simulink library "NG_CHP_lib"  (Simulink 8.1)
settings: Solver=ode45  StartTime=0.0  StopTime=10.0  RelTol=1e-3
undefined symbols (not defined in the file): fdesignblkfcn, gcbh, ph, SIM_HIL, Ts
libraries: simulink x23, rtio_opalrt_common x21, simulink_extras x6, rteventslib x4, CHP_Model_lib x1, NG_Genset_lib x1, rtio_generic_modbus x1
(part 1 of 2)
settings Model: Creator=re25624  LastModifiedBy=re25624

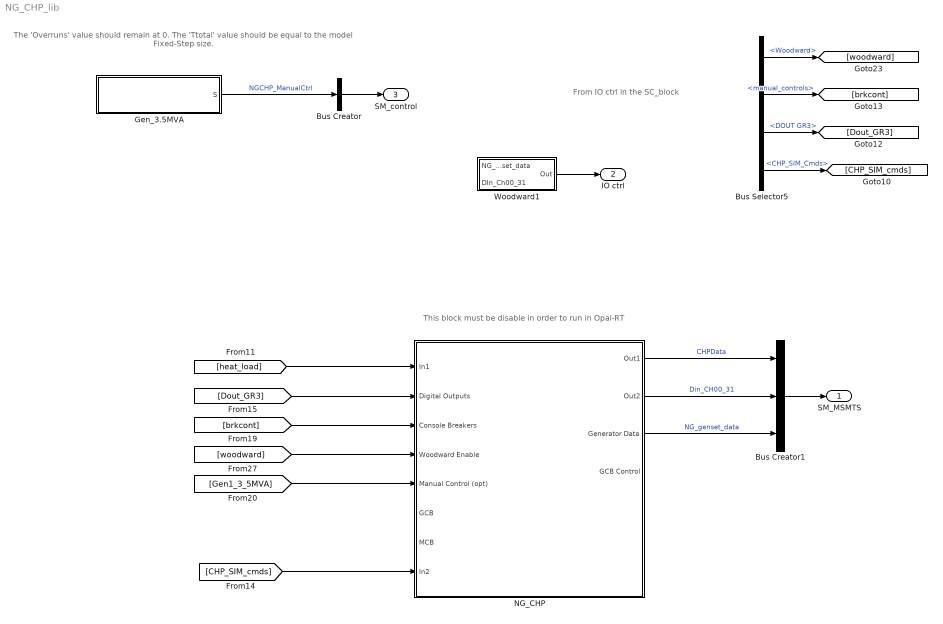
== system NG_CHP_lib ==
  note: From IO ctrl in the SC_block
  note: This block must be disable in order to run in Opal-RT
  note: The 'Overruns' value should remain at 0.
      | The 'Ttotal' value should be equal to the
      | model Fixed-Step size.
  Bus Creator : BusCreator  Inputs=1
  Bus Creator1 : BusCreator  Inputs=3
  Bus Selector5 : BusSelector  OutputSignals=Woodward,manual_controls,DOUT GR3,DOUT GR3.16 DOUT GR3.CHP_SIM_Cmds
  Gen_3.5MVA : Subsystem
  NG_CHP : Subsystem
  Woodward1 : Subsystem
  SM_MSMTS : Outport
  IO ctrl : Outport  Port=2
  SM_control : Outport  Port=3
  wires:
  [Dout_GR3] -> NG_CHP/2(Digital Outputs)
  [brkcont] -> NG_CHP/3(Console Breakers)
  [woodward] -> NG_CHP/4(Woodward Enable)
  [Gen1_3_5MVA] -> NG_CHP/5(Manual Control (opt))
  [heat_load] -> NG_CHP/1(In1)
  Bus Creator1/1 -> SM_MSMTS/1
  NG_CHP/3(Generator Data) -> Bus Creator1/3  "NG_genset_data"
  NG_CHP/2(Out2) -> Bus Creator1/2  "Din_CH00_31"
  NG_CHP/1(Out1) -> Bus Creator1/1  "CHPData"
  [CHP_SIM_cmds] -> NG_CHP/8(In2)
  ? -> Bus Selector5/1
  Bus Selector5/1 -> [woodward]  "<Woodward>"
  Bus Selector5/3 -> [Dout_GR3]  "<DOUT GR3>"
  Bus Selector5/2 -> [brkcont]  "<manual_controls>"
  Bus Selector5/4 -> [CHP_SIM_cmds]  "<CHP_SIM_Cmds>"
  Woodward1/1(Out) -> IO ctrl/1
  Gen_3.5MVA/1(S) -> Bus Creator/1  "NGCHP_ManualCtrl"
  Bus Creator/1 -> SM_control/1

== system NG_CHP_lib/Gen_3.5MVA ==
  1 - PQ 2 - PV 3 - VF : Constant  Value=3
  2.5 - 130 s : DiscretePulseGenerator  Period=150/Ts  PulseWidth=127.5/Ts  PhaseDelay=2.5/Ts  SampleTime=Ts
  Bus Creator : BusCreator  Inputs=6
  DONOTCHANGE : Constant
  Enable = 1 Disable = 0 : Constant  Value=0
  F : simulink/Math Operations/Slider Gain  low=0.97  gain=1  high=1.03
  Fcmd pu : Constant  Value=1.0
  P : simulink/Math Operations/Slider Gain  low=0  gain=0.8  high=1.1
  Pfactor : Gain  Gain=.9
  Q : simulink/Math Operations/Slider Gain  low=0.01  gain=0.2  high=0.4
  Qfactor : Gain  Gain=.43
  S Profile : simulink/Sources/Repeating Sequence Stair  OutValues=[.1 .1 .1 .1 .1 .1 .5 .5 .5 .5 .5 .5 .5 .5 .5 .5 .5 .5 1 1 1 1 1 ]  tsamp=[5 Ts]  OutMin=[]  OutMax=[]  OutDataTypeStr=Inherit: Inherit via back propagation  OutDataType=fixdt(0,8)  ConRadixGroup=Best Precision: Vector-wise  OutScaling=2^-12
  V : simulink/Math Operations/Slider Gain  low=0.9  gain=1  high=1.1
  VF - to end : simulink/Sources/Repeating Sequence Stair  OutValues=[3 3 3 3 3 3 3 3 3 3 3 3 3 3 3 3 3 3 3 3 3 3 3 3 3 3 3 3 3 3 3 ]  tsamp=[5 Ts]  OutMin=[]  OutMax=[]  OutDataTypeStr=Inherit: Inherit via back propagation  OutDataType=fixdt(0,8)  ConRadixGroup=Best Precision: Vector-wise  OutScaling=2^-12
  Vcmd pu : Constant
  S : Outport
  wires:
  DONOTCHANGE/1 -> P/1, Q/1, V/1, F/1
  Bus Creator/1 -> S/1
  S Profile/1 -> Qfactor/1, Pfactor/1  "P"
  Qfactor/1 -> Bus Creator/2  "Q"
  Vcmd pu/1 -> Bus Creator/3  "V"
  VF - to end/1 -> Bus Creator/5  "Mode"
  2.5 - 130 s/1 -> Bus Creator/6  "Enable"
  Fcmd pu/1 -> Bus Creator/4  "F"
  Pfactor/1 -> Bus Creator/1  "P"

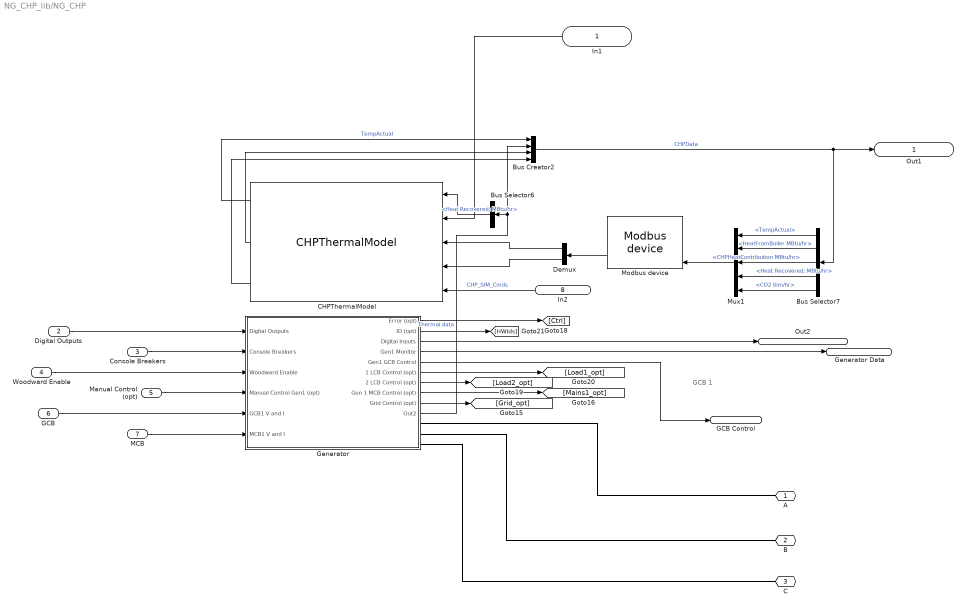
== system NG_CHP_lib/NG_CHP ==
  note: GCB 1
  In1 : Inport
  Digital Outputs : Inport  Port=2
  Console Breakers : Inport  Port=3
  Woodward Enable : Inport  Port=4
  Manual Control (opt) : Inport  Port=5
  GCB : Inport  Port=6
  MCB : Inport  Port=7
  In2 : Inport  Port=8
  Bus Creator2 : BusCreator
  Bus Selector6 : BusSelector  OutputSignals=Heat Recovered; MBtu/hr
  Bus Selector7 : BusSelector  OutputSignals=TempActual,HeatFromBoiler MBtu/hr,CHPHeatContribution MBtu/hr,Thermal data.Heat Recovered; MBtu/hr,Thermal data.CO2 lbm/hr
  CHPThermalModel : CHP_Model_lib/CHPThermalModel  SIM_HIL=SIM_HIL
  Demux : Demux  Outputs=2
  Generator : Subsystem  AncestorBlock=NG_Genset_lib/Generator
  Modbus device : rtio_generic_modbus/Modbus device  conf_name=CHP_slave_cfg.opal  conf_name_mask=CHP_slave_cfg.xls  sample_time=Ts
  Mux1 : Mux  Inputs=5
  A : PMIOPort  Tag=A  Port=1  Side=Right
      settings: AttributesFormatString=A
  B : PMIOPort  Port=2  Side=Right
  C : PMIOPort  Port=3  Side=Right
  Out1 : Outport
  Out2 : Outport  Port=2
  Generator Data : Outport  Port=3
  GCB Control : Outport  Port=4
  wires:
  In2/1 -> CHPThermalModel/5  "CHP_SIM_Cmds"
  Generator/3(Digital Inputs) -> Out2/1
  Bus Creator2/1 -> Out1/1, Bus Selector7/1  "CHPData"
  Bus Selector6/1 -> CHPThermalModel/1  "<Heat Recovered; MBtu/hr>"
  Generator/6(1 LCB Control (opt)) -> [Load1_opt]
  Generator/5(Gen1 GCB Control) -> GCB Control/1
  MCB/1 -> Generator/6(MCB1 V and I)
  Generator/7(2 LCB Control (opt)) -> [Load2_opt]
  Manual Control (opt)/1 -> Generator/4(Manual Control Gen1 (opt))
  GCB/1 -> Generator/5(GCB1 V and I)
  Generator/4(Gen1 Monitor) -> Generator Data/1
  Generator/1(Error (opt)) -> [Ctrl]
  Woodward Enable/1 -> Generator/3(Woodward Enable)
  Generator/2(ID (opt)) -> [HWIds]
  Modbus device/2 -> Demux/1
  Generator/10(Out2) -> Bus Selector6/1, Bus Creator2/2  "Thermal data"
  CHPThermalModel/3 -> Bus Creator2/4
  Demux/1 -> CHPThermalModel/3
  Mux1/1 -> Modbus device/4
  In1/1 -> CHPThermalModel/2
  Bus Selector7/1 -> Mux1/1  "<TempActual>"
  Bus Selector7/4 -> Mux1/4  "<Heat Recovered; MBtu/hr>"
  Bus Selector7/5 -> Mux1/5  "<CO2 lbm/hr>"
  Bus Selector7/2 -> Mux1/2  "<HeatFromBoiler MBtu/hr>"
  Digital Outputs/1 -> Generator/1(Digital Outputs)
  Generator/9(Grid Control (opt)) -> [Grid_opt]
  Console Breakers/1 -> Generator/2(Console Breakers)
  Generator/8(Gen 1 MCB Control (opt)) -> [Mains1_opt]
  CHPThermalModel/2 -> Bus Creator2/3
  Demux/2 -> CHPThermalModel/4
  CHPThermalModel/1 -> Bus Creator2/1  "TempActual"
  Bus Selector7/3 -> Mux1/3  "<CHPHeatContribution MBtu/hr>"
  connections:
  Generator/RConn1 -- A/RConn1
  Generator/RConn2 -- B/RConn1
  Generator/RConn3 -- C/RConn1

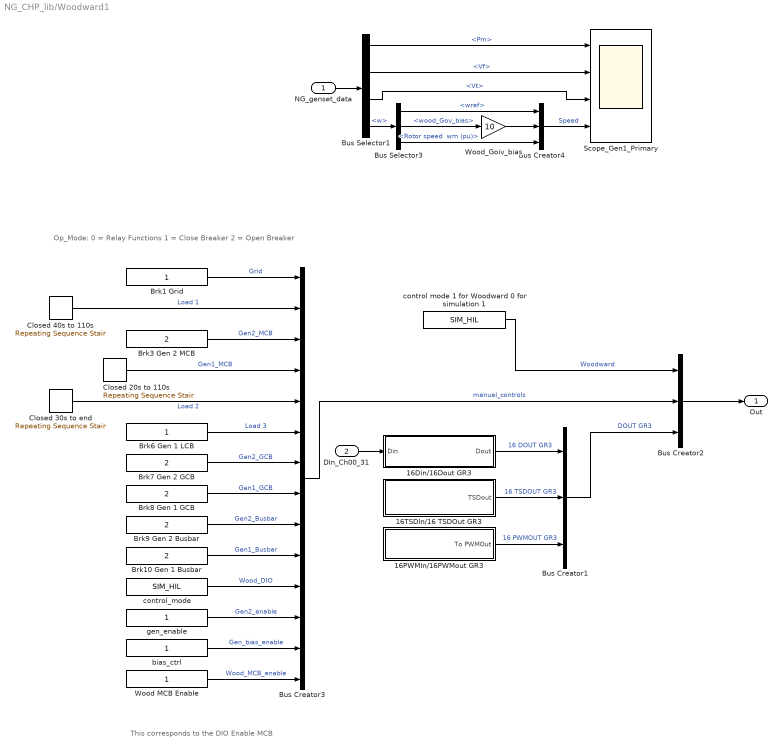
== system NG_CHP_lib/Woodward1 ==
  note: Op_Mode:
      | 0 = Relay Functions
      | 1 = Close Breaker
      | 2 = Open Breaker
  note: This corresponds to
      | the DIO Enable MCB
  NG_genset_data : Inport
  DIn_Ch00_31 : Inport  Port=2
  16Din/16Dout GR3 : Subsystem
  16PWMIn/16PWMout GR3 : Subsystem
  16TSDIn/16 TSDOut GR3 : Subsystem
  Brk1 Grid : Constant
  Brk10 Gen 1 Busbar : Constant  Value=2
  Brk3 Gen 2 MCB : Constant  Value=2
  Brk6 Gen 1 LCB : Constant
  Brk7 Gen 2 GCB : Constant  Value=2
  Brk8 Gen 1 GCB : Constant  Value=2
  Brk9 Gen 2 Busbar : Constant  Value=2
  Bus Creator1 : BusCreator  Inputs=3
  Bus Creator2 : BusCreator  Inputs=3
  Bus Creator3 : BusCreator  Inputs=14
  Bus Creator4 : BusCreator  Inputs=3
  Bus Selector1 : BusSelector  OutputSignals=Pm,Vf,Vt,w
  Bus Selector3 : BusSelector  OutputSignals="wref,w.wood_Gov_bias,w.Rotor speed  wm (pu)"
  Closed 20s to 110s : simulink/Sources/Repeating Sequence Stair  OutValues=[2 2 2 2 1 1 1 1 1 1 1 1 1 1 1 1 1 1 1 1 1 1 2 2 2 2 2]  tsamp=[5 Ts]  OutMin=[]  OutMax=[]  OutDataTypeStr=double  OutputDataTypeScalingMode=double  OutDataType=fixdt(0,8)  ConRadixGroup=Best Precision: Vector-wise  OutScaling=2^-12
  Closed 30s to end : simulink/Sources/Repeating Sequence Stair  OutValues=[2 2 2 2 2 2 1 1 1 1 1 1 1 1 1 1 1 1 1 1 1 1 ]  tsamp=[5 Ts]  OutMin=[]  OutMax=[]  OutDataTypeStr=double  OutputDataTypeScalingMode=double  OutDataType=fixdt(0,8)  ConRadixGroup=Best Precision: Vector-wise  OutScaling=2^-12
  Closed 40s to 110s : simulink/Sources/Repeating Sequence Stair  OutValues=[2 2 2 2 2 2 2 2 1 1 1 1 1 1 1 1 1 1 1 1 1 1 2 2 2]  tsamp=[5 Ts]  OutMin=[]  OutMax=[]  OutDataTypeStr=double  OutputDataTypeScalingMode=double  OutDataType=fixdt(0,8)  ConRadixGroup=Best Precision: Vector-wise  OutScaling=2^-12
  Scope_Gen1_Primary : Scope  NumInputPorts=4
      settings: TimeRange=10  YMin=-0.05~-0.5~0~0  YMax=0.8~5.5~1.1~1.1  SaveName=ScopeData4
  Wood MCB Enable : Constant
  Wood_Goiv_bias : Gain  Gain=10
  bias_ctrl : Constant
  control mode 1 for Woodward 0 for simulation 1 : Constant  Value=SIM_HIL
  control_mode : Constant  Value=SIM_HIL
  gen_enable : Constant
  Out : Outport
  wires:
  control mode 1 for Woodward 0 for simulation 1/1 -> Bus Creator2/1  "Woodward"
  16Din/16Dout GR3/1(Dout) -> Bus Creator1/1  "16 DOUT GR3"
  16TSDIn/16 TSDOut GR3/1(TSDout) -> Bus Creator1/2  "16 TSDOUT GR3"
  16PWMIn/16PWMout GR3/1(To PWMOut) -> Bus Creator1/3  "16 PWMOUT GR3"
  Bus Creator1/1 -> Bus Creator2/3  "DOUT GR3"
  Bus Creator3/1 -> Bus Creator2/2  "manual_controls"
  Closed 40s to 110s/1 -> Bus Creator3/2  "Load 1"
  Brk3 Gen 2 MCB/1 -> Bus Creator3/3  "Gen2_MCB"
  Closed 20s to 110s/1 -> Bus Creator3/4  "Gen1_MCB"
  control_mode/1 -> Bus Creator3/11  "Wood_DIO"
  gen_enable/1 -> Bus Creator3/12  "Gen2_enable"
  bias_ctrl/1 -> Bus Creator3/13  "Gen_bias_enable"
  Bus Creator2/1 -> Out/1
  DIn_Ch00_31/1 -> 16Din/16Dout GR3/1(Din)
  Bus Selector1/1 -> Scope_Gen1_Primary/1  "<Pm>"
  Bus Selector1/2 -> Scope_Gen1_Primary/2  "<Vf>"
  Bus Selector1/3 -> Scope_Gen1_Primary/3  "<Vt>"
  NG_genset_data/1 -> Bus Selector1/1
  Wood MCB Enable/1 -> Bus Creator3/14  "Wood_MCB_enable"
  Bus Selector1/4 -> Bus Selector3/1  "<w>"
  Bus Selector3/1 -> Bus Creator4/1  "<wref>"
  Bus Selector3/2 -> Wood_Goiv_bias/1  "<wood_Gov_bias>"
  Bus Selector3/3 -> Bus Creator4/3  "<Rotor speed  wm (pu)>"
  Bus Creator4/1 -> Scope_Gen1_Primary/4  "Speed"
  Closed 30s to end/1 -> Bus Creator3/5  "Load 2"
  Brk6 Gen 1 LCB/1 -> Bus Creator3/6  "Load 3"
  Brk7 Gen 2 GCB/1 -> Bus Creator3/7  "Gen2_GCB"
  Brk8 Gen 1 GCB/1 -> Bus Creator3/8  "Gen1_GCB"
  Wood_Goiv_bias/1 -> Bus Creator4/2
  Brk9 Gen 2 Busbar/1 -> Bus Creator3/9  "Gen2_Busbar"
  Brk10 Gen 1 Busbar/1 -> Bus Creator3/10  "Gen1_Busbar"
  Brk1 Grid/1 -> Bus Creator3/1  "Grid"

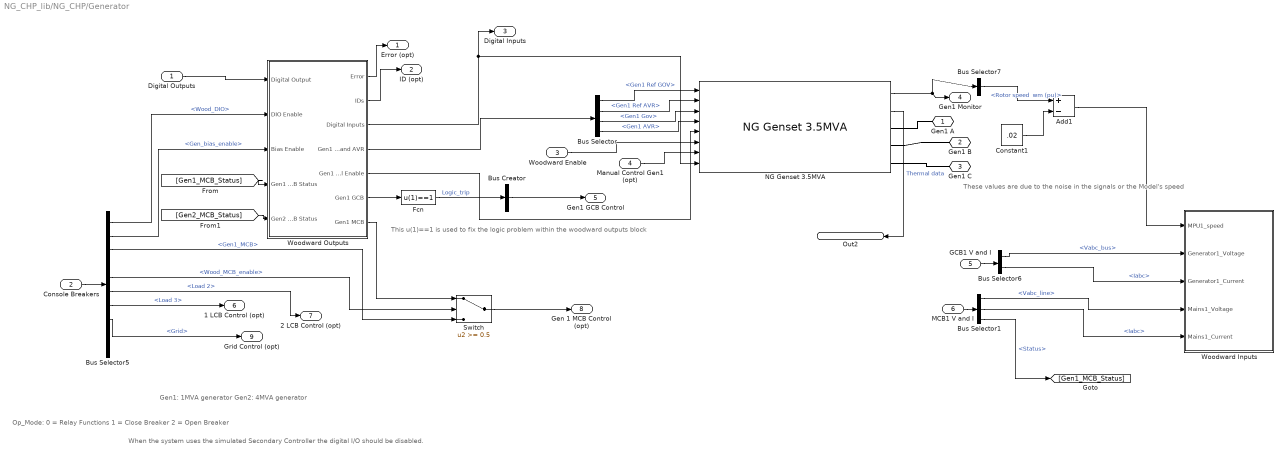
== system NG_CHP_lib/NG_CHP/Generator ==
  note: Op_Mode:
      | 0 = Relay Functions
      | 1 = Close Breaker
      | 2 = Open Breaker
  note: These values are due to
      | the noise in the signals
      | or the Model's speed
  note: Gen1: 1MVA generator
      | Gen2: 4MVA generator
  note: When the system uses the simulated
      | Secondary Controller the digital I/O
      | should be disabled.
  note: This u(1)==1 is used to fix the logic problem within the woodward outputs block
  Digital Outputs : Inport
  Console Breakers : Inport  Port=2
  Woodward Enable : Inport  Port=3
  Manual Control Gen1 (opt) : Inport  Port=4
  GCB1 V and I : Inport  Port=5
  MCB1 V and I : Inport  Port=6
  Add1 : Sum  Inputs=+-
  Bus Creator : BusCreator  Inputs=1
  Bus Selector : BusSelector  OutputSignals=Gen1 Ref GOV,Gen1 Ref AVR,Gen1 Gov,Gen1 AVR
  Bus Selector1 : BusSelector  OutputSignals=Vabc_line,Iabc,Status
  Bus Selector5 : BusSelector  OutputSignals=Wood_DIO,Gen_bias_enable,Gen1_MCB,Gen2_MCB,Wood_MCB_enable,Load 2,Load 3,Grid,Gen2_enable,Load 1
  Bus Selector6 : BusSelector  OutputSignals=Vabc_bus,Iabc
  Bus Selector7 : BusSelector  OutputSignals="w.w.Rotor speed  wm (pu)"
  Constant1 : Constant  Value=.02
  Fcn : Fcn  Expr=u(1)==1
  NG Genset 3.5MVA : NG_Genset_lib/NG Genset 3.5MVA  control_mode=1
  Switch : Switch  Threshold=0.5
  Woodward Inputs : Subsystem
  Woodward Outputs : Subsystem
  Gen1 A : PMIOPort  Port=1  Side=Right
  Gen1 B : PMIOPort  Port=2  Side=Right
  Gen1 C : PMIOPort  Port=3  Side=Right
  Error (opt) : Outport
  ID (opt) : Outport  Port=2
  Digital Inputs : Outport  Port=3
  Gen1 Monitor : Outport  Port=4
  Gen1 GCB Control : Outport  Port=5
  1 LCB Control (opt) : Outport  Port=6
  2 LCB Control (opt) : Outport  Port=7
  Gen 1 MCB Control (opt) : Outport  Port=8
  Grid Control (opt) : Outport  Port=9
  Out2 : Outport  Port=10
  wires:
  Fcn/1 -> Bus Creator/1  "Logic_trip"
  Bus Creator/1 -> Gen1 GCB Control/1
  NG Genset 3.5MVA/1 -> Bus Selector7/1, Gen1 Monitor/1
  Bus Selector6/1 -> Woodward Inputs/2(Generator1_Voltage)  "<Vabc_bus>"
  Bus Selector6/2 -> Woodward Inputs/3(Generator1_Current)  "<Iabc>"
  Bus Selector5/1 -> Woodward Outputs/2(DIO Enable)  "<Wood_DIO>"
  Manual Control Gen1 (opt)/1 -> NG Genset 3.5MVA/7
  Bus Selector5/2 -> Woodward Outputs/3(Bias Enable)  "<Gen_bias_enable>"
  Bus Selector7/1 -> Add1/1  "<Rotor speed  wm (pu)>"
  Woodward Outputs/1(Error) -> Error (opt)/1
  Woodward Outputs/2(IDs) -> ID (opt)/1
  Woodward Enable/1 -> NG Genset 3.5MVA/6
  Woodward Outputs/5(Gen1 Fuel Enable) -> NG Genset 3.5MVA/5
  Bus Selector5/5 -> Switch/2  "<Wood_MCB_enable>"
  Woodward Outputs/7(Gen1 MCB) -> Switch/1
  Digital Outputs/1 -> Woodward Outputs/1(Digital Output)
  GCB1 V and I/1 -> Bus Selector6/1
  Woodward Outputs/6(Gen1 GCB) -> Fcn/1
  Console Breakers/1 -> Bus Selector5/1
  Bus Selector5/7 -> 1 LCB Control (opt)/1  "<Load 3>"
  Switch/1 -> Gen 1 MCB Control (opt)/1
  MCB1 V and I/1 -> Bus Selector1/1
  Bus Selector1/1 -> Woodward Inputs/4(Mains1_Voltage)  "<Vabc_line>"
  Bus Selector1/2 -> Woodward Inputs/5(Mains1_Current)  "<Iabc>"
  Woodward Outputs/4(Gen1 Gov and AVR) -> Bus Selector/1
  Bus Selector/1 -> NG Genset 3.5MVA/1  "<Gen1 Ref GOV>"
  Bus Selector/2 -> NG Genset 3.5MVA/2  "<Gen1 Ref AVR>"
  Bus Selector/3 -> NG Genset 3.5MVA/3  "<Gen1 Gov>"
  Bus Selector/4 -> NG Genset 3.5MVA/4  "<Gen1 AVR>"
  Bus Selector1/3 -> [Gen1_MCB_Status]  "<Status>"
  [Gen1_MCB_Status] -> Woodward Outputs/4(Gen1 MCB Status)
  [Gen2_MCB_Status] -> Woodward Outputs/5(Gen2 MCB Status)
  Bus Selector5/6 -> 2 LCB Control (opt)/1  "<Load 2>"
  Bus Selector5/3 -> Switch/3  "<Gen1_MCB>"
  Bus Selector5/8 -> Grid Control (opt)/1  "<Grid>"
  Constant1/1 -> Add1/2
  NG Genset 3.5MVA/2 -> Out2/1  "Thermal data"
  Add1/1 -> Woodward Inputs/1(MPU1_speed)
  Woodward Outputs/3(Digital Inputs) -> Digital Inputs/1, NG Genset 3.5MVA/8
  connections:
  NG Genset 3.5MVA/RConn1 -- Gen1 A/RConn1
  NG Genset 3.5MVA/RConn2 -- Gen1 B/RConn1
  NG Genset 3.5MVA/RConn3 -- Gen1 C/RConn1

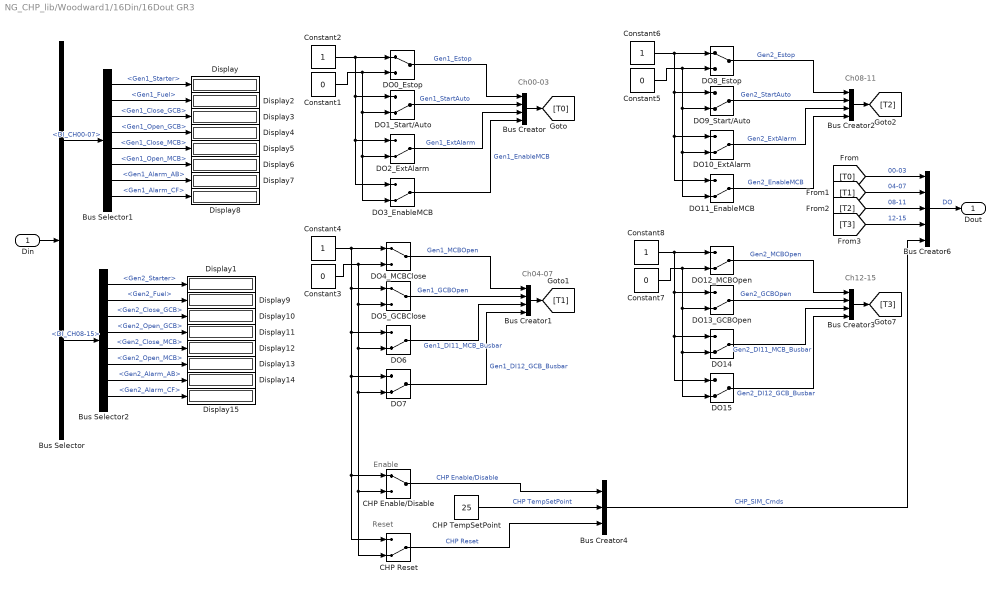
== system NG_CHP_lib/Woodward1/16Din/16Dout GR3 ==
  note: Ch00-03
  note: Ch04-07
  note: Ch08-11
  note: Ch12-15
  note: Enable
  note: Reset
  Din : Inport
  Bus Creator{,1..3} (4 alike) : BusCreator
  Bus Creator4 : BusCreator  Inputs=3
  Bus Creator6 : BusCreator  Inputs=5
  Bus Selector : BusSelector  OutputSignals=DIN.DI_CH00-07,DIN.DI_CH08-15
  Bus Selector1 : BusSelector  OutputSignals=Gen1_Starter,Gen1_Fuel,Gen1_Close_GCB,Gen1_Open_GCB,Gen1_Close_MCB,Gen1_Open_MCB,Gen1_Alarm_AB,Gen1_Alarm_CF
  Bus Selector2 : BusSelector  OutputSignals=Gen2_Starter,Gen2_Fuel,Gen2_Close_GCB,Gen2_Open_GCB,Gen2_Close_MCB,Gen2_Open_MCB,Gen2_Alarm_AB,Gen2_Alarm_CF
  CHP Enable/Disable : ManualSwitch
  CHP Reset : ManualSwitch  CurrentSetting=0
  CHP TempSetPoint : Constant  Value=25
  Constant{1,3,5,7} (4 alike) : Constant  Value=0
  Constant{2,4,6,8} (4 alike) : Constant
  DO0_Estop : ManualSwitch
  DO10_ExtAlarm : ManualSwitch  CurrentSetting=0
  DO11_EnableMCB : ManualSwitch  CurrentSetting=0
  DO12_MCBOpen : ManualSwitch  CurrentSetting=0
  DO13_GCBOpen : ManualSwitch  CurrentSetting=0
  DO{6..7,14..15} (4 alike) : ManualSwitch  CurrentSetting=0
  DO1_Start/Auto : ManualSwitch  CurrentSetting=0
  DO2_ExtAlarm : ManualSwitch  CurrentSetting=0
  DO3_EnableMCB : ManualSwitch  CurrentSetting=0
  DO4_MCBClose : ManualSwitch
  DO5_GCBClose : ManualSwitch
  DO8_Estop : ManualSwitch
  DO9_Start/Auto : ManualSwitch  CurrentSetting=0
  Display{,1..15} (16 alike) : Display
  Dout : Outport
  wires:
  Bus Creator4/1 -> Bus Creator6/5  "CHP_SIM_Cmds"
  CHP Reset/1 -> Bus Creator4/3  "CHP Reset"
  CHP TempSetPoint/1 -> Bus Creator4/2  "CHP TempSetPoint"
  CHP Enable/Disable/1 -> Bus Creator4/1  "CHP Enable/Disable"
  Bus Creator6/1 -> Dout/1  "DO"
  Constant2/1 -> DO0_Estop/1, DO1_Start/Auto/1, DO3_EnableMCB/1, DO2_ExtAlarm/1
  Constant1/1 -> DO0_Estop/2, DO1_Start/Auto/2, DO3_EnableMCB/2, DO2_ExtAlarm/2
  DO0_Estop/1 -> Bus Creator/1  "Gen1_Estop"
  DO1_Start/Auto/1 -> Bus Creator/2  "Gen1_StartAuto"
  DO2_ExtAlarm/1 -> Bus Creator/3  "Gen1_ExtAlarm"
  DO3_EnableMCB/1 -> Bus Creator/4  "Gen1_EnableMCB"
  Constant4/1 -> DO6/1, DO7/1, CHP Enable/Disable/1, CHP Reset/1, DO5_GCBClose/1, DO4_MCBClose/1
  Constant3/1 -> DO6/2, CHP Enable/Disable/2, CHP Reset/2, DO7/2, DO5_GCBClose/2, DO4_MCBClose/2
  DO4_MCBClose/1 -> Bus Creator1/1  "Gen1_MCBOpen"
  DO5_GCBClose/1 -> Bus Creator1/2  "Gen1_GCBOpen"
  DO6/1 -> Bus Creator1/3  "Gen1_DI11_MCB_Busbar"
  DO7/1 -> Bus Creator1/4  "Gen1_DI12_GCB_Busbar"
  Constant6/1 -> DO8_Estop/1, DO9_Start/Auto/1, DO11_EnableMCB/1, DO10_ExtAlarm/1
  Constant5/1 -> DO8_Estop/2, DO9_Start/Auto/2, DO11_EnableMCB/2, DO10_ExtAlarm/2
  DO8_Estop/1 -> Bus Creator2/1  "Gen2_Estop"
  DO9_Start/Auto/1 -> Bus Creator2/2  "Gen2_StartAuto"
  DO10_ExtAlarm/1 -> Bus Creator2/3  "Gen2_ExtAlarm"
  DO11_EnableMCB/1 -> Bus Creator2/4  "Gen2_EnableMCB"
  Constant8/1 -> DO14/1, DO15/1, DO13_GCBOpen/1, DO12_MCBOpen/1
  Constant7/1 -> DO14/2, DO15/2, DO13_GCBOpen/2, DO12_MCBOpen/2
  DO12_MCBOpen/1 -> Bus Creator3/1  "Gen2_MCBOpen"
  DO13_GCBOpen/1 -> Bus Creator3/2  "Gen2_GCBOpen"
  DO14/1 -> Bus Creator3/3  "Gen2_DI11_MCB_Busbar"
  DO15/1 -> Bus Creator3/4  "Gen2_DI12_GCB_Busbar"
  Bus Creator/1 -> [T0]
  Bus Creator1/1 -> [T1]
  Bus Creator3/1 -> [T3]
  Bus Creator2/1 -> [T2]
  [T0] -> Bus Creator6/1  "00-03"
  [T1] -> Bus Creator6/2  "04-07"
  [T2] -> Bus Creator6/3  "08-11"
  [T3] -> Bus Creator6/4  "12-15"
  Din/1 -> Bus Selector/1
  Bus Selector/1 -> Bus Selector1/1  "<DI_CH00-07>"
  Bus Selector1/1 -> Display/1  "<Gen1_Starter>"
  Bus Selector1/2 -> Display2/1  "<Gen1_Fuel>"
  Bus Selector1/3 -> Display3/1  "<Gen1_Close_GCB>"
  Bus Selector1/5 -> Display5/1  "<Gen1_Close_MCB>"
  Bus Selector1/6 -> Display6/1  "<Gen1_Open_MCB>"
  Bus Selector1/8 -> Display8/1  "<Gen1_Alarm_CF>"
  Bus Selector/2 -> Bus Selector2/1  "<DI_CH08-15>"
  Bus Selector2/1 -> Display1/1  "<Gen2_Starter>"
  Bus Selector2/2 -> Display9/1  "<Gen2_Fuel>"
  Bus Selector2/3 -> Display10/1  "<Gen2_Close_GCB>"
  Bus Selector2/4 -> Display11/1  "<Gen2_Open_GCB>"
  Bus Selector2/5 -> Display12/1  "<Gen2_Close_MCB>"
  Bus Selector2/6 -> Display13/1  "<Gen2_Open_MCB>"
  Bus Selector2/7 -> Display14/1  "<Gen2_Alarm_AB>"
  Bus Selector2/8 -> Display15/1  "<Gen2_Alarm_CF>"
  Bus Selector1/4 -> Display4/1  "<Gen1_Open_GCB>"
  Bus Selector1/7 -> Display7/1  "<Gen1_Alarm_AB>"

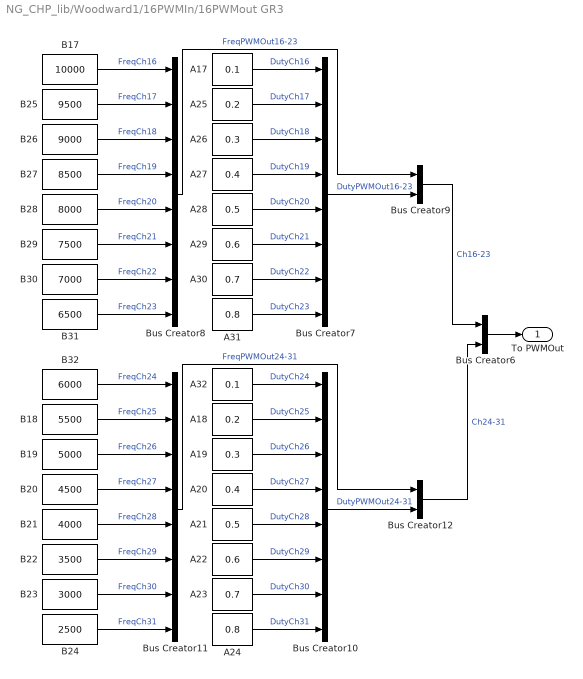
== system NG_CHP_lib/Woodward1/16PWMIn/16PWMout GR3 ==
  A17 : Constant  Value=0.1
  A18 : Constant  Value=0.2
  A19 : Constant  Value=0.3
  A20 : Constant  Value=0.4
  A21 : Constant  Value=0.5
  A22 : Constant  Value=0.6
  A23 : Constant  Value=0.7
  A24 : Constant  Value=0.8
  A25 : Constant  Value=0.2
  A26 : Constant  Value=0.3
  A27 : Constant  Value=0.4
  A28 : Constant  Value=0.5
  A29 : Constant  Value=0.6
  A30 : Constant  Value=0.7
  A31 : Constant  Value=0.8
  A32 : Constant  Value=0.1
  B17 : Constant  Value=10000
  B18 : Constant  Value=5500
  B19 : Constant  Value=5000
  B20 : Constant  Value=4500
  B21 : Constant  Value=4000
  B22 : Constant  Value=3500
  B23 : Constant  Value=3000
  B24 : Constant  Value=2500
  B25 : Constant  Value=9500
  B26 : Constant  Value=9000
  B27 : Constant  Value=8500
  B28 : Constant  Value=8000
  B29 : Constant  Value=7500
  B30 : Constant  Value=7000
  B31 : Constant  Value=6500
  B32 : Constant  Value=6000
  Bus Creator{7..8,10..11} (4 alike) : BusCreator  Inputs=8
  Bus Creator12 : BusCreator  Inputs=2
  Bus Creator6 : BusCreator  Inputs=2
  Bus Creator9 : BusCreator  Inputs=2
  To PWMOut : Outport
  wires:
  Bus Creator6/1 -> To PWMOut/1
  A17/1 -> Bus Creator7/1  "DutyCh16"
  A25/1 -> Bus Creator7/2  "DutyCh17"
  A26/1 -> Bus Creator7/3  "DutyCh18"
  A27/1 -> Bus Creator7/4  "DutyCh19"
  A28/1 -> Bus Creator7/5  "DutyCh20"
  A29/1 -> Bus Creator7/6  "DutyCh21"
  A30/1 -> Bus Creator7/7  "DutyCh22"
  A31/1 -> Bus Creator7/8  "DutyCh23"
  B17/1 -> Bus Creator8/1  "FreqCh16"
  B25/1 -> Bus Creator8/2  "FreqCh17"
  B26/1 -> Bus Creator8/3  "FreqCh18"
  B27/1 -> Bus Creator8/4  "FreqCh19"
  B28/1 -> Bus Creator8/5  "FreqCh20"
  B29/1 -> Bus Creator8/6  "FreqCh21"
  B30/1 -> Bus Creator8/7  "FreqCh22"
  B31/1 -> Bus Creator8/8  "FreqCh23"
  Bus Creator7/1 -> Bus Creator9/2  "DutyPWMOut16-23"
  Bus Creator8/1 -> Bus Creator9/1  "FreqPWMOut16-23"
  A32/1 -> Bus Creator10/1  "DutyCh24"
  A18/1 -> Bus Creator10/2  "DutyCh25"
  A19/1 -> Bus Creator10/3  "DutyCh26"
  A20/1 -> Bus Creator10/4  "DutyCh27"
  A21/1 -> Bus Creator10/5  "DutyCh28"
  A22/1 -> Bus Creator10/6  "DutyCh29"
  A23/1 -> Bus Creator10/7  "DutyCh30"
  A24/1 -> Bus Creator10/8  "DutyCh31"
  B32/1 -> Bus Creator11/1  "FreqCh24"
  B18/1 -> Bus Creator11/2  "FreqCh25"
  B19/1 -> Bus Creator11/3  "FreqCh26"
  B20/1 -> Bus Creator11/4  "FreqCh27"
  B21/1 -> Bus Creator11/5  "FreqCh28"
  B22/1 -> Bus Creator11/6  "FreqCh29"
  B23/1 -> Bus Creator11/7  "FreqCh30"
  B24/1 -> Bus Creator11/8  "FreqCh31"
  Bus Creator10/1 -> Bus Creator12/2  "DutyPWMOut24-31"
  Bus Creator11/1 -> Bus Creator12/1  "FreqPWMOut24-31"
  Bus Creator12/1 -> Bus Creator6/2  "Ch24-31"
  Bus Creator9/1 -> Bus Creator6/1  "Ch16-23"

== system NG_CHP_lib/Woodward1/16TSDIn/16 TSDOut GR3 ==
  Bus Creator1 : BusCreator  Inputs=3
  Din/Dout ch16-23 : Subsystem
  Din/Dout ch24-31 : Subsystem
  Dout state ctrl : Subsystem
  TSDout : Outport
  wires:
  Din/Dout ch24-31/1(Out1) -> Bus Creator1/2  "times CH24-31"
  Din/Dout ch16-23/1(Out1) -> Bus Creator1/1  "times CH16-23"
  Dout state ctrl/1(Event State OUT) -> Bus Creator1/3  "states"
  Bus Creator1/1 -> TSDout/1

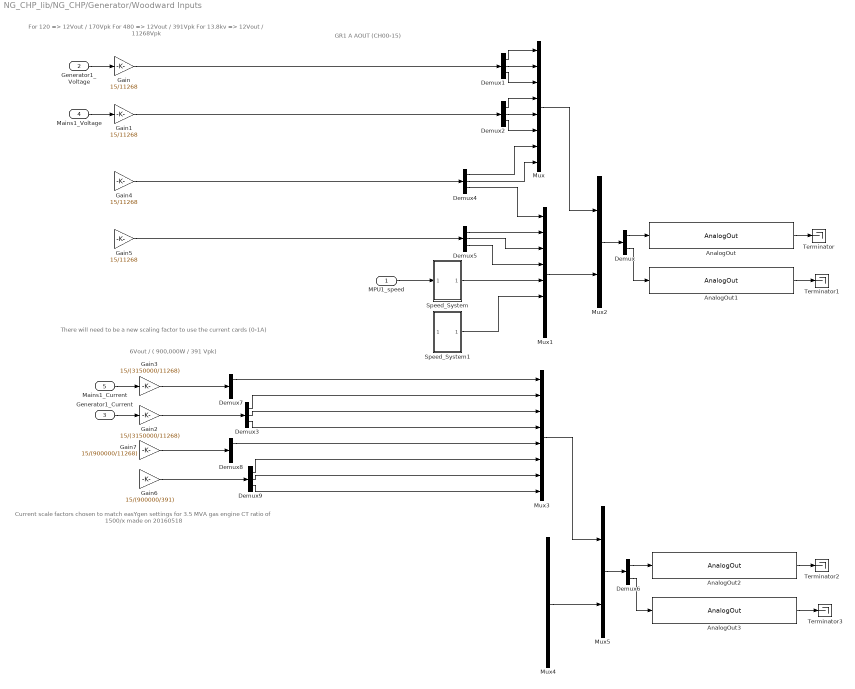
== system NG_CHP_lib/NG_CHP/Generator/Woodward Inputs ==
  note: Current scale factors chosen to match
      | easYgen settings for 3.5 MVA gas engine
      | CT ratio of 1500/x made on 20160518
  note: 6Vout / ( 900,000W / 391 Vpk)
  note: For 120 => 12Vout / 170Vpk
      | For 480 => 12Vout / 391Vpk
      | For 13.8kv => 12Vout / 11268Vpk
  note: GR1 A AOUT (CH00-15)
  note: There will need to be a
      | new scaling factor to use
      | the current cards (0-1A)
  MPU1_speed : Inport
  Generator1_Voltage : Inport  Port=2
  Generator1_Current : Inport  Port=3
  Mains1_Voltage : Inport  Port=4
  Mains1_Current : Inport  Port=5
  AnalogOut : rtio_opalrt_common/AnalogOut  CtrlName='OpCtrl'  portNb=1  FcnNos=Slot 1 Module A Subsection 1  size=16  maxcount=-2  count=-2  numchan=-2  israngeinput=off  voltagerange=[-16 ... 16]  slot=0  side=0  mismatch=0  slotside=Slot_1_Module_A
      settings: AttributesFormatString=%<CtrlName>
  AnalogOut1 : rtio_opalrt_common/AnalogOut  CtrlName='OpCtrl'  portNb=2  FcnNos=Slot 1 Module A Subsection 2  size=16  maxcount=-2  count=-2  numchan=-2  israngeinput=off  voltagerange=[-16 ... 16]  slot=0  side=0  mismatch=0  slotside=Slot_1_Module_A
      settings: AttributesFormatString=%<CtrlName>
  AnalogOut2 : rtio_opalrt_common/AnalogOut  CtrlName='OpCtrl'  portNb=3  FcnNos=Slot 2 Module A Subsection 1  size=16  maxcount=-2  count=-2  numchan=-2  israngeinput=off  voltagerange=[-16 ... 16]  slot=1  side=0  mismatch=0  slotside=Slot_2_Module_A
      settings: AttributesFormatString=%<CtrlName>
  AnalogOut3 : rtio_opalrt_common/AnalogOut  CtrlName='OpCtrl'  portNb=4  FcnNos=Slot 2 Module A Subsection 2  size=16  maxcount=-2  count=-2  numchan=-2  israngeinput=off  voltagerange=[-16 ... 16]  slot=1  side=0  mismatch=0  slotside=Slot_2_Module_A
      settings: AttributesFormatString=%<CtrlName>
  Demux : Demux  Outputs=2
  Demux{1..5,7..9} (8 alike) : Demux  Outputs=3
  Demux6 : Demux  Outputs=2
  Gain{,1,4..5} (4 alike) : Gain  Gain=15/11268
  Gain2 : Gain  Gain=15/(3150000/11268)
  Gain3 : Gain  Gain=15/(3150000/11268)
  Gain6 : Gain  Gain=15/(900000/391)
  Gain7 : Gain  Gain=15/(900000/11268)
  Mux{,1,3..4} (4 alike) : Mux  Inputs=8
  Mux2 : Mux  Inputs=2
  Mux5 : Mux  Inputs=2
  Speed_System : Subsystem
  Speed_System1 : Subsystem
  Terminator{,1..3} (4 alike) : Terminator
  wires:
  MPU1_speed/1 -> Speed_System/1(In1)
  Generator1_Current/1 -> Gain2/1
  Gain1/1 -> Demux2/1
  Gain/1 -> Demux1/1
  Mains1_Voltage/1 -> Gain1/1
  Mux2/1 -> Demux/1
  Mux1/1 -> Mux2/2
  Mux/1 -> Mux2/1
  Generator1_Voltage/1 -> Gain/1
  Demux/2 -> AnalogOut1/1
  Demux/1 -> AnalogOut/1
  AnalogOut1/1 -> Terminator1/1
  AnalogOut/1 -> Terminator/1
  Demux1/1 -> Mux/1
  Demux1/2 -> Mux/2
  Demux1/3 -> Mux/3
  Demux2/1 -> Mux/4
  Demux2/2 -> Mux/5
  Demux2/3 -> Mux/6
  Speed_System/1(Out1) -> Mux1/5
  Demux4/1 -> Mux/7
  Demux4/2 -> Mux/8
  Demux4/3 -> Mux1/1
  Demux5/1 -> Mux1/2
  Demux5/2 -> Mux1/3
  Demux5/3 -> Mux1/4
  Mux5/1 -> Demux6/1
  Mux4/1 -> Mux5/2
  Mux3/1 -> Mux5/1
  Demux6/2 -> AnalogOut3/1
  Demux6/1 -> AnalogOut2/1
  AnalogOut3/1 -> Terminator3/1
  AnalogOut2/1 -> Terminator2/1
  Gain2/1 -> Demux3/1
  Demux3/1 -> Mux3/2
  Demux3/2 -> Mux3/3
  Demux3/3 -> Mux3/4
  Mains1_Current/1 -> Gain3/1
  Gain3/1 -> Demux7/1
  Demux7/1 -> Mux3/1
  Gain5/1 -> Demux5/1
  Gain4/1 -> Demux4/1
  ? -> Gain5/1
  ? -> Gain4/1
  ? -> Speed_System1/1(In1)
  Speed_System1/1(Out1) -> Mux1/6
  ? -> Gain6/1
  ? -> Gain7/1
  Gain7/1 -> Demux8/1
  Demux8/1 -> Mux3/5
  Gain6/1 -> Demux9/1
  Demux9/1 -> Mux3/6
  Demux9/2 -> Mux3/7
  Demux9/3 -> Mux3/8

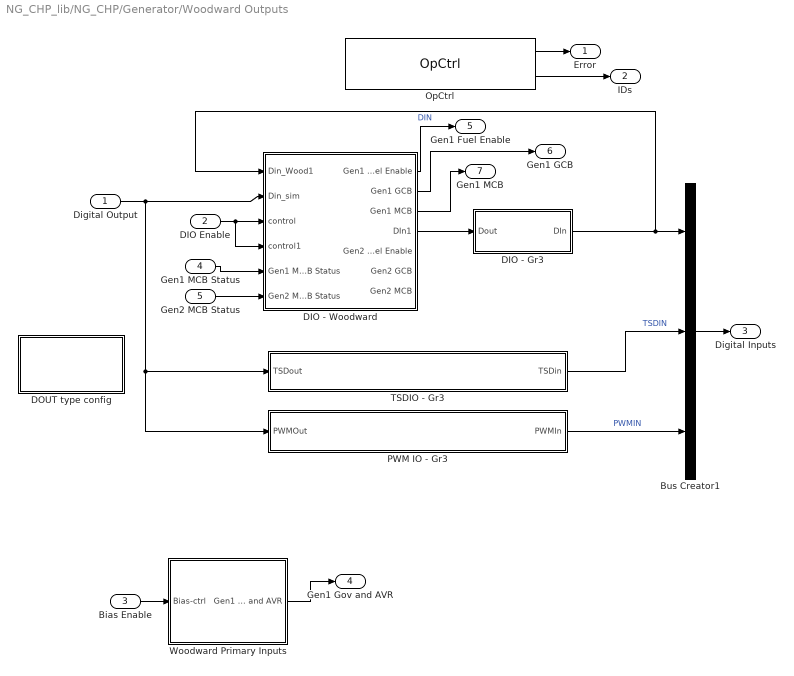
== system NG_CHP_lib/NG_CHP/Generator/Woodward Outputs ==
  Digital Output : Inport
  DIO Enable : Inport  Port=2
  Bias Enable : Inport  Port=3
  Gen1 MCB Status : Inport  Port=4
  Gen2 MCB Status : Inport  Port=5
  Bus Creator1 : BusCreator  Inputs=3
  DIO - Gr3 : Subsystem
  DIO - Woodward : Subsystem
  DOUT type config : Subsystem
  OpCtrl : rtio_opalrt_common/OpCtrl  CtrlName='OpCtrl'  boardid=0  BitstreamFilename=VC707_2-EX-0001-2_2_6_61-32AIO16DIO16DIOSel-01-01.bin  numconfig=-1  mode=Master  externalClock=off  decimRtsi=0  calibIO=off  SampleTime=0  loadinport=-1  BoardType=VC707  SecondaryPresent=off  sync_type=Audio
  PWM IO - Gr3 : Subsystem
  TSDIO - Gr3 : Subsystem
  Woodward Primary Inputs : Subsystem
  Error : Outport
  IDs : Outport  Port=2
  Digital Inputs : Outport  Port=3
  Gen1 Gov and AVR : Outport  Port=4
  Gen1 Fuel Enable : Outport  Port=5
  Gen1 GCB : Outport  Port=6
  Gen1 MCB : Outport  Port=7
  wires:
  OpCtrl/1 -> Error/1
  OpCtrl/2 -> IDs/1
  DIO - Woodward/4(DIn1) -> DIO - Gr3/1(Dout)
  PWM IO - Gr3/1(PWMIn) -> Bus Creator1/3  "PWMIN"
  TSDIO - Gr3/1(TSDin) -> Bus Creator1/2  "TSDIN"
  DIO - Gr3/1(DIn) -> Bus Creator1/1, DIO - Woodward/1(Din_Wood1)  "DIN"
  Bus Creator1/1 -> Digital Inputs/1
  DIO Enable/1 -> DIO - Woodward/3(control), DIO - Woodward/4(control1)
  Woodward Primary Inputs/1(Gen1 Gov and AVR) -> Gen1 Gov and AVR/1
  Bias Enable/1 -> Woodward Primary Inputs/1(Bias-ctrl)
  Digital Output/1 -> DIO - Woodward/2(Din_sim), PWM IO - Gr3/1(PWMOut), TSDIO - Gr3/1(TSDout)
  DIO - Woodward/2(Gen1 GCB) -> Gen1 GCB/1
  DIO - Woodward/3(Gen1 MCB) -> Gen1 MCB/1
  DIO - Woodward/1(Gen1 Fuel Enable) -> Gen1 Fuel Enable/1
  Gen1 MCB Status/1 -> DIO - Woodward/5(Gen1 MCB Status)
  Gen2 MCB Status/1 -> DIO - Woodward/6(Gen2 MCB Status)

== system NG_CHP_lib/Woodward1/16TSDIn/16 TSDOut GR3/Din/Dout ch16-23 ==
  Bus Creator3 : BusCreator  Inputs=8
  times17 : Constant  Value=[0.05 0.15 0.25 0.35]
  times18 : Constant  Value=[0.1 0.2 0.3 0.4]
  times19 : Constant  Value=[0.15 0.25 0.35 0.45]
  times20 : Constant  Value=[0.2 0.3 0.4 0.5]
  times21 : Constant  Value=[0.25 0.35 0.45 0.55]
  times22 : Constant  Value=[0.3 0.4 0.5 0.6]
  times23 : Constant  Value=[0.3 0.4 0.5 0.6]
  times24 : Constant  Value=[0 0.1 0.2 0.3]
  Out1 : Outport
  wires:
  Bus Creator3/1 -> Out1/1
  times23/1 -> Bus Creator3/8  "times24"
  times22/1 -> Bus Creator3/7  "times23"
  times21/1 -> Bus Creator3/6  "times22"
  times20/1 -> Bus Creator3/5  "times21"
  times19/1 -> Bus Creator3/4  "times20"
  times18/1 -> Bus Creator3/3  "times19"
  times17/1 -> Bus Creator3/2  "times18"
  times24/1 -> Bus Creator3/1  "times17"

== system NG_CHP_lib/Woodward1/16TSDIn/16 TSDOut GR3/Din/Dout ch24-31 ==
  Bus Creator4 : BusCreator  Inputs=8
  times25 : Constant  Value=[0.05 0.15 0.25 0.35]
  times26 : Constant  Value=[0.1 0.2 0.3 0.4]
  times27 : Constant  Value=[0.15 0.25 0.35 0.45]
  times28 : Constant  Value=[0.2 0.3 0.4 0.5]
  times29 : Constant  Value=[0.25 0.35 0.45 0.55]
  times30 : Constant  Value=[0.3 0.4 0.5 0.6]
  times31 : Constant  Value=[0.3 0.4 0.5 0.6]
  times32 : Constant  Value=[0 0.1 0.2 0.3]
  Out1 : Outport
  wires:
  Bus Creator4/1 -> Out1/1
  times31/1 -> Bus Creator4/8  "times32"
  times30/1 -> Bus Creator4/7  "times31"
  times29/1 -> Bus Creator4/6  "times30"
  times28/1 -> Bus Creator4/5  "times29"
  times27/1 -> Bus Creator4/4  "times28"
  times26/1 -> Bus Creator4/3  "times27"
  times25/1 -> Bus Creator4/2  "times26"
  times32/1 -> Bus Creator4/1  "times25"

== system NG_CHP_lib/Woodward1/16TSDIn/16 TSDOut GR3/Dout state ctrl ==
  Bus Creator : BusCreator  Inputs=2
  Dout_CH16_CH23 : Subsystem
  Dout_CH24_CH31 : Subsystem
  Event State OUT : Outport
  wires:
  Dout_CH24_CH31/1(Dout_CH8_CH15) -> Bus Creator/2  "CH24-31"
  Dout_CH16_CH23/1(Dout_CH8_CH15) -> Bus Creator/1  "CH16-23"
  Bus Creator/1 -> Event State OUT/1

== system NG_CHP_lib/NG_CHP/Generator/Woodward Inputs/Speed_System ==
  In1 : Inport
  Clock1 : Clock
      settings: DisableCoverage=on
  Duty : Constant  DisableCoverage=on  Value=0.5
  Gain1 : Gain  Gain=5
  Gain3 : Gain  Gain=5
  Gain4 : Gain  Gain=1800
  Output : Trigonometry
  Product1 : Product  DisableCoverage=on  SaturateOnIntegerOverflow=on  InputSameDT=on  OutDataTypeStr=Inherit: Same as first input
  Product3 : Product  DisableCoverage=on  SaturateOnIntegerOverflow=on  InputSameDT=on  OutDataTypeStr=Inherit: Same as first input
  RTE Conversion : rteventslib/Signal Attributes/RTE Conversion  inputdatatype=RTE Boolean  outputdatatype=Double  compensation=Disabled  nbMaxEvents=10  sampleTime=Ts
  RTE SPWM : rteventslib/Sources/RTE SPWM  NumberPhases=1-ph  CenterAlignmentMode=On  MaxFreq=inf  MinFreq=0  EnablingPort=off  ComplementaryMode=off  SpaceVector=off  RiseTimeDelay=0  MaxEvents=10  SampleTime=Ts
  initialFreq : Constant  DisableCoverage=on  Value=2*pi
  Out1 : Outport
  wires:
  Gain1/1 -> Out1/1
  RTE Conversion/1 -> Gain1/1
  Duty/1 -> RTE SPWM/2
  RTE SPWM/1 -> RTE Conversion/1
  In1/1 -> Gain4/1
  Output/1 -> Gain3/1
  Gain4/1 -> RTE SPWM/1, Product3/2
  Product3/1 -> Product1/2
  initialFreq/1 -> Product3/1
  Clock1/1 -> Product1/1
  Product1/1 -> Output/1

== system NG_CHP_lib/NG_CHP/Generator/Woodward Inputs/Speed_System1 ==
  In1 : Inport
  Clock1 : Clock
      settings: DisableCoverage=on
  Duty : Constant  DisableCoverage=on  Value=0.5
  Gain1 : Gain  Gain=5
  Gain3 : Gain  Gain=5
  Gain4 : Gain  Gain=1800
  Output : Trigonometry
  Product1 : Product  DisableCoverage=on  SaturateOnIntegerOverflow=on  InputSameDT=on  OutDataTypeStr=Inherit: Same as first input
  Product3 : Product  DisableCoverage=on  SaturateOnIntegerOverflow=on  InputSameDT=on  OutDataTypeStr=Inherit: Same as first input
  RTE Conversion : rteventslib/Signal Attributes/RTE Conversion  inputdatatype=RTE Boolean  outputdatatype=Double  compensation=Disabled  nbMaxEvents=10  sampleTime=Ts
  RTE SPWM : rteventslib/Sources/RTE SPWM  NumberPhases=1-ph  CenterAlignmentMode=On  MaxFreq=inf  MinFreq=0  EnablingPort=off  ComplementaryMode=off  SpaceVector=off  RiseTimeDelay=0  MaxEvents=10  SampleTime=Ts
  initialFreq : Constant  DisableCoverage=on  Value=2*pi
  Out1 : Outport
  wires:
  Gain1/1 -> Out1/1
  RTE Conversion/1 -> Gain1/1
  Duty/1 -> RTE SPWM/2
  RTE SPWM/1 -> RTE Conversion/1
  In1/1 -> Gain4/1
  Output/1 -> Gain3/1
  Gain4/1 -> RTE SPWM/1, Product3/2
  Product3/1 -> Product1/2
  initialFreq/1 -> Product3/1
  Clock1/1 -> Product1/1
  Product1/1 -> Output/1

== system NG_CHP_lib/NG_CHP/Generator/Woodward Outputs/DIO - Gr3 ==
  Dout : Inport
  Bus Creator : BusCreator  Inputs=2
  Bus Selector : BusSelector  OutputSignals=DI_CH00-07  OutputAsBus=on
  Bus Selector1 : BusSelector  OutputSignals=DI_CH08-15  OutputAsBus=on
  Conditioning : Subsystem
  Conditioning1 : Subsystem
  DigitalIn : rtio_opalrt_common/DigitalIn  CtrlName='OpCtrl'  portNb=5  FcnNos=Slot 3 Module A Subsection 1  size=1  maxcount=-2  count=-2  sampleTime=0  numchan=-2
      settings: AttributesFormatString=%<CtrlName>
  DigitalIn1 : rtio_opalrt_common/DigitalIn  CtrlName='OpCtrl'  portNb=6  FcnNos=Slot 3 Module A Subsection 2  size=1  maxcount=-2  count=-2  sampleTime=0  numchan=-2
      settings: AttributesFormatString=%<CtrlName>
  DigitalOut : rtio_opalrt_common/DigitalOut  CtrlName='OpCtrl'  portNb=5  FcnNos=Slot 3 Module B Subsection 1  size=1  maxcount=-2  count=8  numchan=8
      settings: AttributesFormatString=%<CtrlName>
  DigitalOut1 : rtio_opalrt_common/DigitalOut  CtrlName='OpCtrl'  portNb=6  FcnNos=Slot 3 Module B Subsection 2  size=1  maxcount=-2  count=8  numchan=8
      settings: AttributesFormatString=%<CtrlName>
  Terminator{1,3,5..6} (4 alike) : Terminator
  DIn : Outport
  wires:
  DigitalOut/1 -> Terminator3/1
  DigitalOut1/1 -> Terminator1/1
  Dout/1 -> Bus Selector/1, Bus Selector1/1
  Bus Selector/1 -> DigitalOut/1
  Bus Selector1/1 -> DigitalOut1/1
  DigitalIn/2 -> Terminator5/1
  DigitalIn1/2 -> Terminator6/1
  DigitalIn/1 -> Conditioning/1(In1)  "DI_CH00-07"
  DigitalIn1/1 -> Conditioning1/1(In1)  "DI_CH08-15"
  Bus Creator/1 -> DIn/1
  Conditioning/1(Out1) -> Bus Creator/1
  Conditioning1/1(Out1) -> Bus Creator/2

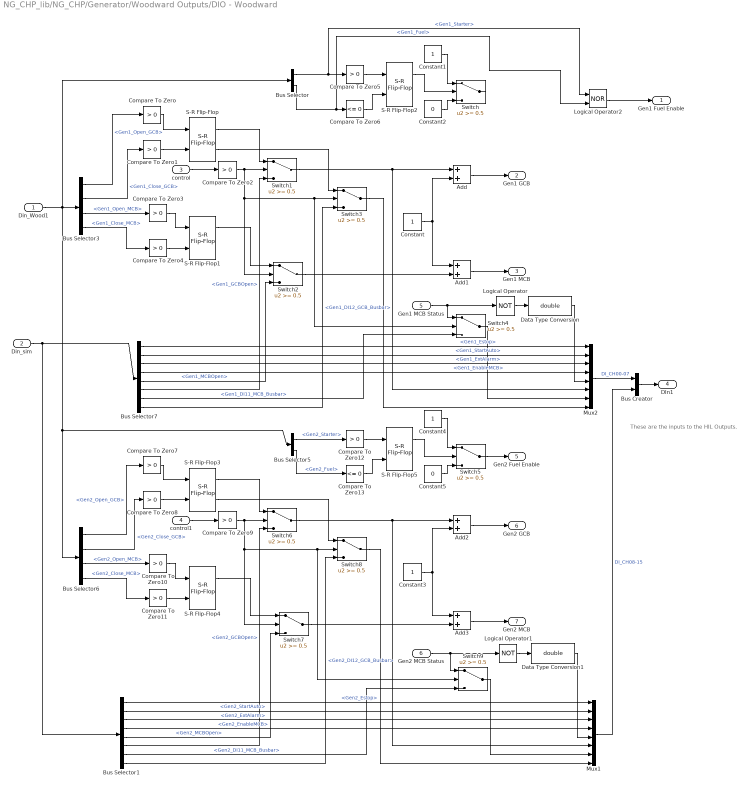
== system NG_CHP_lib/NG_CHP/Generator/Woodward Outputs/DIO - Woodward ==
  note: These are the inputs to
      | the HIL Outputs.
  Din_Wood1 : Inport
  Din_sim : Inport  Port=2
  control : Inport  Port=3
  control1 : Inport  Port=4
  Gen1 MCB Status : Inport  Port=5
  Gen2 MCB Status : Inport  Port=6
  Add{,1..3} (4 alike) : Sum
  Bus Creator : BusCreator  Inputs=2
  Bus Selector : BusSelector  OutputSignals=DI_CH00-07.Gen1_Starter,DI_CH00-07.Gen1_Fuel
  Bus Selector1 : BusSelector  OutputSignals=16 DOUT GR3.08-11.Gen2_Estop,16 DOUT GR3.08-11.Gen2_StartAuto,16 DOUT GR3.08-11.Gen2_ExtAlarm,16 DOUT GR3.08-11.Gen2_EnableMCB,16 DOUT GR3.12-15.Gen2_MCBOpen,16 DOUT GR3.12-15.Gen2_GCBOpen,16 DOUT GR3.12-15.Gen2_DI11_MCB_Busbar,16 DOUT GR3.12-15.Gen2_DI12_GCB_Busbar
  Bus Selector3 : BusSelector  OutputSignals=DI_CH00-07.Gen1_Open_GCB,DI_CH00-07.Gen1_Close_GCB,DI_CH00-07.Gen1_Open_MCB,DI_CH00-07.Gen1_Close_MCB
  Bus Selector5 : BusSelector  OutputSignals=DI_CH08-15.Gen2_Starter,DI_CH08-15.Gen2_Fuel
  Bus Selector6 : BusSelector  OutputSignals=DI_CH08-15.Gen2_Open_GCB,DI_CH08-15.Gen2_Close_GCB,DI_CH08-15.Gen2_Open_MCB,DI_CH08-15.Gen2_Close_MCB
  Bus Selector7 : BusSelector  OutputSignals=16 DOUT GR3.00-03.Gen1_Estop,16 DOUT GR3.00-03.Gen1_StartAuto,16 DOUT GR3.00-03.Gen1_ExtAlarm,16 DOUT GR3.00-03.Gen1_EnableMCB,16 DOUT GR3.04-07.Gen1_MCBOpen,16 DOUT GR3.04-07.Gen1_GCBOpen,16 DOUT GR3.04-07.Gen1_DI11_MCB_Busbar,16 DOUT GR3.04-07.Gen1_DI12_GCB_Busbar
  Compare To Zero{,1..5,7..12} (12 alike) : simulink/Logic and Bit Operations/Compare To Zero  relop=>  OutDataTypeStr=boolean
  Compare To Zero13 : simulink/Logic and Bit Operations/Compare To Zero  relop=<=  OutDataTypeStr=boolean
  Compare To Zero6 : simulink/Logic and Bit Operations/Compare To Zero  relop=<=  OutDataTypeStr=boolean
  Constant{,1,3..4} (4 alike) : Constant
  Constant2 : Constant  Value=0
  Constant5 : Constant  Value=0
  Data Type Conversion : DataTypeConversion  OutDataTypeStr=double
  Data Type Conversion1 : DataTypeConversion  OutDataTypeStr=double
  Logical Operator : Logic  Operator=NOT  AllPortsSameDT=off  OutDataTypeStr=boolean
  Logical Operator1 : Logic  Operator=NOT  AllPortsSameDT=off  OutDataTypeStr=boolean
  Logical Operator2 : Logic  Operator=NOR  AllPortsSameDT=off  OutDataTypeStr=boolean
  Mux1 : Mux  Inputs=8
  Mux2 : Mux  Inputs=8
  S-R Flip-Flop{,1,3..4} (4 alike) : simulink_extras/Flip Flops/S-R Flip-Flop  initial_condition=1
  S-R Flip-Flop2 : simulink_extras/Flip Flops/S-R Flip-Flop  initial_condition=0
  S-R Flip-Flop5 : simulink_extras/Flip Flops/S-R Flip-Flop  initial_condition=0
  Switch : Switch  Threshold=0.5
  Switch{1..4,6..9} (8 alike) : Switch  Threshold=0.5  OutDataTypeStr=double
      Switch8 settings: LockScale=on
  Switch5 : Switch  Threshold=0.5
  Gen1 Fuel Enable : Outport
  Gen1 GCB : Outport  Port=2
  Gen1 MCB : Outport  Port=3
  DIn1 : Outport  Port=4
  Gen2 Fuel Enable : Outport  Port=5
  Gen2 GCB : Outport  Port=6
  Gen2 MCB : Outport  Port=7
  wires:
  Bus Selector3/2 -> Compare To Zero1/1  "<Gen1_Close_GCB>"
  Bus Selector3/1 -> Compare To Zero/1  "<Gen1_Open_GCB>"
  Din_Wood1/1 -> Bus Selector3/1, Bus Selector/1, Bus Selector6/1, Bus Selector5/1
  control/1 -> Compare To Zero2/1
  Bus Creator/1 -> DIn1/1
  S-R Flip-Flop/1 -> Switch1/1
  Switch1/1 -> Add/1, Mux2/6
  Compare To Zero/1 -> S-R Flip-Flop/1
  Compare To Zero1/1 -> S-R Flip-Flop/2
  Bus Selector3/4 -> Compare To Zero4/1  "<Gen1_Close_MCB>"
  Compare To Zero4/1 -> S-R Flip-Flop1/2
  Compare To Zero3/1 -> S-R Flip-Flop1/1
  S-R Flip-Flop1/1 -> Switch2/1
  Compare To Zero2/1 -> Switch1/2, Switch2/2, Switch3/2, Switch4/2
  Switch2/1 -> Add1/2
  Mux1/1 -> Bus Creator/2  "DI_CH08-15"
  S-R Flip-Flop/2 -> Switch3/1
  Add/1 -> Gen1 GCB/1
  Add1/1 -> Gen1 MCB/1
  Constant/1 -> Add/2, Add1/1
  Bus Selector/1 -> Logical Operator2/1, Compare To Zero5/1  "<Gen1_Starter>"
  Bus Selector/2 -> Logical Operator2/2, Compare To Zero6/1  "<Gen1_Fuel>"
  S-R Flip-Flop2/1 -> Switch/2
  Compare To Zero5/1 -> S-R Flip-Flop2/1
  Constant2/1 -> Switch/3
  Constant1/1 -> Switch/1
  Compare To Zero6/1 -> S-R Flip-Flop2/2
  control1/1 -> Compare To Zero9/1
  S-R Flip-Flop3/1 -> Switch6/1
  Switch6/1 -> Add2/1, Mux1/6
  Bus Selector6/1 -> Compare To Zero7/1  "<Gen2_Open_GCB>"
  Compare To Zero7/1 -> S-R Flip-Flop3/1
  Compare To Zero8/1 -> S-R Flip-Flop3/2
  Bus Selector6/4 -> Compare To Zero11/1  "<Gen2_Close_MCB>"
  Compare To Zero11/1 -> S-R Flip-Flop4/2
  Bus Selector6/3 -> Compare To Zero10/1  "<Gen2_Open_MCB>"
  Compare To Zero10/1 -> S-R Flip-Flop4/1
  S-R Flip-Flop4/1 -> Switch7/1
  Bus Selector6/2 -> Compare To Zero8/1  "<Gen2_Close_GCB>"
  Compare To Zero9/1 -> Switch6/2, Switch7/2, Switch8/2, Switch9/2
  Switch7/1 -> Add3/2
  S-R Flip-Flop3/2 -> Switch8/1
  Add2/1 -> Gen2 GCB/1
  Add3/1 -> Gen2 MCB/1
  Constant3/1 -> Add2/2, Add3/1
  Bus Selector5/1 -> Compare To Zero12/1  "<Gen2_Starter>"
  Bus Selector5/2 -> Compare To Zero13/1  "<Gen2_Fuel>"
  S-R Flip-Flop5/1 -> Switch5/2
  Compare To Zero12/1 -> S-R Flip-Flop5/1
  Constant5/1 -> Switch5/3
  Constant4/1 -> Switch5/1
  Compare To Zero13/1 -> S-R Flip-Flop5/2
  Switch5/1 -> Gen2 Fuel Enable/1
  Bus Selector3/3 -> Compare To Zero3/1  "<Gen1_Open_MCB>"
  Bus Selector1/1 -> Mux1/1  "<Gen2_Estop>"
  Bus Selector1/2 -> Mux1/2  "<Gen2_StartAuto>"
  Bus Selector1/3 -> Mux1/3  "<Gen2_ExtAlarm>"
  Bus Selector1/4 -> Mux1/4  "<Gen2_EnableMCB>"
  Bus Selector1/5 -> Switch7/3  "<Gen2_MCBOpen>"
  Bus Selector1/6 -> Switch6/3  "<Gen2_GCBOpen>"
  Bus Selector7/1 -> Mux2/1  "<Gen1_Estop>"
  Bus Selector7/2 -> Mux2/2  "<Gen1_StartAuto>"
  Bus Selector7/3 -> Mux2/3  "<Gen1_ExtAlarm>"
  Bus Selector7/4 -> Mux2/4  "<Gen1_EnableMCB>"
  Bus Selector7/5 -> Switch2/3  "<Gen1_MCBOpen>"
  Bus Selector7/6 -> Switch1/3  "<Gen1_GCBOpen>"
  Mux2/1 -> Bus Creator/1  "DI_CH00-07"
  Din_sim/1 -> Bus Selector7/1, Bus Selector1/1
  Bus Selector7/7 -> Switch4/3  "<Gen1_DI11_MCB_Busbar>"
  Switch4/1 -> Mux2/7
  Bus Selector7/8 -> Switch3/3  "<Gen1_DI12_GCB_Busbar>"
  Switch3/1 -> Mux2/8
  Bus Selector1/7 -> Switch9/3  "<Gen2_DI11_MCB_Busbar>"
  Switch9/1 -> Mux1/7
  Bus Selector1/8 -> Switch8/3  "<Gen2_DI12_GCB_Busbar>"
  Switch8/1 -> Mux1/8
  Gen1 MCB Status/1 -> Logical Operator/1, Switch4/1
  Data Type Conversion/1 -> Mux2/5
  Logical Operator/1 -> Data Type Conversion/1
  Gen2 MCB Status/1 -> Logical Operator1/1, Switch9/1
  Logical Operator1/1 -> Data Type Conversion1/1
  Data Type Conversion1/1 -> Mux1/5
  Logical Operator2/1 -> Gen1 Fuel Enable/1

== system NG_CHP_lib/NG_CHP/Generator/Woodward Outputs/DOUT type config ==
  note: The Constants are used to select Digital Output type:
      | - 0: Time-Stamped Digital Output
      | - 1: Pulse-Width Modulated DIgital Output
  DataIn Send : rtio_opalrt_common/DataIn Send  CtrlName='OpCtrl'  FcnNos=11  width=1  portType=double  checkVersion=off  expectedId=0  expectedVersion=0  opComp=>=
      settings: AttributesFormatString=%<CtrlName>
  DataIn Send1 : rtio_opalrt_common/DataIn Send  CtrlName='OpCtrl'  FcnNos=12  width=1  portType=double  checkVersion=off  expectedId=0  expectedVersion=0  opComp=>=
      settings: AttributesFormatString=%<CtrlName>
  Subsection 3 DOUT type : Constant
  Subsection 4 DOUT type : Constant
  Terminator1 : Terminator
  Terminator2 : Terminator
  wires:
  Subsection 3 DOUT type/1 -> DataIn Send/1
  Subsection 4 DOUT type/1 -> DataIn Send1/1
  DataIn Send1/1 -> Terminator1/1
  DataIn Send/1 -> Terminator2/1

== system NG_CHP_lib/NG_CHP/Generator/Woodward Outputs/PWM IO - Gr3 ==
  PWMOut : Inport
  Bus Creator : BusCreator  Inputs=2
  Bus Creator1 : BusCreator  Inputs=2
  Bus Creator2 : BusCreator  Inputs=2
  Bus Selector : BusSelector  OutputSignals=FreqPWMOut16-23,DutyPWMOut16-23
  Bus Selector1 : BusSelector  OutputSignals=FreqPWMOut24-31,DutyPWMOut24-31
  Bus Selector2 : BusSelector  OutputSignals=16 PWMOUT GR3.Ch16-23,16 PWMOUT GR3.Ch24-31
  PWM In : rtio_opalrt_common/PWM In  CtrlName='OpCtrl'  portNb=9  FcnNos=Slot 3 Module A Subsection 3  maxCount=8  Count=8  sampleTime=0  numchan=8
      settings: AttributesFormatString=%<CtrlName>
  PWM In1 : rtio_opalrt_common/PWM In  CtrlName='OpCtrl'  portNb=10  FcnNos=Slot 3 Module A Subsection 4  maxCount=8  Count=8  sampleTime=0  numchan=8
      settings: AttributesFormatString=%<CtrlName>
  PWM Out : rtio_opalrt_common/PWM Out  CtrlName='OpCtrl'  portNb=9  FcnNos=Slot 3 Module B Subsection 3  size=64  maxcount=8  count=8  polarity=Active High  symMode=Symmetric  complementary=off  deadTime=0  numchan=8  loadnb=1  initphase=[0 0 0 0 0 0 0 0]
      settings: AttributesFormatString=%<CtrlName>
  PWM Out1 : rtio_opalrt_common/PWM Out  CtrlName='OpCtrl'  portNb=10  FcnNos=Slot 3 Module B Subsection 4  size=64  maxcount=8  count=8  polarity=Active High  symMode=Symmetric  complementary=off  deadTime=0  numchan=8  loadnb=2  initphase=[0 0 0 0 0 0 0 0]
      settings: AttributesFormatString=%<CtrlName>
  Terminator{,1,4..5} (4 alike) : Terminator
  PWMIn : Outport
  wires:
  Bus Selector/1 -> PWM Out/1  "<FreqPWMOut16-23>"
  Bus Selector/2 -> PWM Out/2  "<DutyPWMOut16-23>"
  PWM Out/1 -> Terminator/1
  Bus Selector1/1 -> PWM Out1/1  "<FreqPWMOut24-31>"
  Bus Selector1/2 -> PWM Out1/2  "<DutyPWMOut24-31>"
  PWM Out1/1 -> Terminator1/1
  PWMOut/1 -> Bus Selector2/1
  Bus Selector2/1 -> Bus Selector/1  "<Ch16-23>"
  Bus Creator/1 -> PWMIn/1
  Bus Creator1/1 -> Bus Creator/1  "PWMI_CH16-23"
  Bus Creator2/1 -> Bus Creator/2  "PWMI_CH24-31"
  PWM In1/3 -> Terminator5/1
  PWM In/3 -> Terminator4/1
  PWM In/1 -> Bus Creator1/1  "Freq"
  PWM In/2 -> Bus Creator1/2  "Duty"
  PWM In1/1 -> Bus Creator2/1  "Freq"
  PWM In1/2 -> Bus Creator2/2  "Duty"
  Bus Selector2/2 -> Bus Selector1/1  "<Ch24-31>"

== system NG_CHP_lib/NG_CHP/Generator/Woodward Outputs/TSDIO - Gr3 ==
  TSDout : Inport
  Bus Creator : BusCreator  Inputs=16
  Bus Creator1 : BusCreator  Inputs=16
  Bus Creator2 : BusCreator  Inputs=2
  Bus Selector : BusSelector  OutputSignals=16 TSDOUT GR3.states.CH16-23.states 17,16 TSDOUT GR3.times CH16-23.times17,16 TSDOUT GR3.states.CH16-23.states 18,16 TSDOUT GR3.times CH16-23.times18,16 TSDOUT GR3.states.CH16-23.states 19,16 TSDOUT GR3.times CH16-23.times19,16 TSDOUT GR3.states.CH16-23.states 20,16 TSDOUT GR3.times CH16-23.times20,16 TSDOUT GR3.states.CH16-23.states 21,16 TSDOUT GR3.times CH16-23.times21,16 TSDOUT GR3.states.CH16-23.states 22,16 TSDOUT GR3.times CH16-23.times22,16 TSDOUT GR3.states.CH16-23.states 23,16 TSDOUT GR3.times CH16-23.times23,16 TSDOUT GR3.states.CH16-23.states 24,16 TSDOUT GR3.times CH16-23.times24
  Bus Selector1 : BusSelector  OutputSignals=16 TSDOUT GR3.states.CH24-31.states 25,16 TSDOUT GR3.times CH24-31.times25,16 TSDOUT GR3.states.CH24-31.states 26,16 TSDOUT GR3.times CH24-31.times26,16 TSDOUT GR3.states.CH24-31.states 27,16 TSDOUT GR3.times CH24-31.times27,16 TSDOUT GR3.states.CH24-31.states 28,16 TSDOUT GR3.times CH24-31.times28,16 TSDOUT GR3.states.CH24-31.states 29,16 TSDOUT GR3.times CH24-31.times29,16 TSDOUT GR3.states.CH24-31.states 30,16 TSDOUT GR3.times CH24-31.times30,16 TSDOUT GR3.states.CH24-31.states 31,16 TSDOUT GR3.times CH24-31.times31,16 TSDOUT GR3.states.CH24-31.states 32,16 TSDOUT GR3.times CH24-31.times32
  EventDetector : rtio_opalrt_common/EventDetector  CtrlName='OpCtrl'  portNb=7  FcnNos=Slot 3 Module A Subsection 3  size=32  maxcount=-2  nbChannels=8  width=4  timeUnit=Time ratio  sampleTime=0  numwidth=4
      settings: AttributesFormatString=%<CtrlName>
  EventDetector1 : rtio_opalrt_common/EventDetector  CtrlName='OpCtrl'  portNb=8  FcnNos=Slot 3 Module A Subsection 4  size=32  maxcount=-2  nbChannels=8  width=4  timeUnit=Time ratio  sampleTime=0  numwidth=4
      settings: AttributesFormatString=%<CtrlName>
  EventGenerator : rtio_opalrt_common/EventGenerator  CtrlName='OpCtrl'  portNb=7  FcnNos=Slot 3 Module B Subsection 3  size=32  count=8  nbChannels=8  width=4  timeUnit=Time ratio  numwidth=4
      settings: AttributesFormatString=%<CtrlName>
  EventGenerator1 : rtio_opalrt_common/EventGenerator  CtrlName='OpCtrl'  portNb=8  FcnNos=Slot 3 Module B Subsection 4  size=32  count=8  nbChannels=8  width=4  timeUnit=Time ratio  numwidth=4
      settings: AttributesFormatString=%<CtrlName>
  Terminator{,1..3} (4 alike) : Terminator
  TSDin : Outport
  wires:
  TSDout/1 -> Bus Selector/1, Bus Selector1/1
  Bus Selector/16 -> EventGenerator/16  "<times24>"
  Bus Selector/15 -> EventGenerator/15  "<states 24>"
  Bus Selector/14 -> EventGenerator/14  "<times23>"
  Bus Selector/13 -> EventGenerator/13  "<states 23>"
  Bus Selector/12 -> EventGenerator/12  "<times22>"
  Bus Selector/11 -> EventGenerator/11  "<states 22>"
  Bus Selector/10 -> EventGenerator/10  "<times21>"
  Bus Selector/9 -> EventGenerator/9  "<states 21>"
  Bus Selector/8 -> EventGenerator/8  "<times20>"
  Bus Selector/7 -> EventGenerator/7  "<states 20>"
  Bus Selector/6 -> EventGenerator/6  "<times19>"
  Bus Selector/5 -> EventGenerator/5  "<states 19>"
  Bus Selector/4 -> EventGenerator/4  "<times18>"
  Bus Selector/3 -> EventGenerator/3  "<states 18>"
  Bus Selector/2 -> EventGenerator/2  "<times17>"
  Bus Selector/1 -> EventGenerator/1  "<states 17>"
  EventGenerator/1 -> Terminator/1
  EventDetector/16 -> Bus Creator/16  "times8"
  EventDetector/15 -> Bus Creator/15  "states8"
  EventDetector/14 -> Bus Creator/14  "times7"
  EventDetector/13 -> Bus Creator/13  "states7"
  EventDetector/12 -> Bus Creator/12  "times6"
  EventDetector/11 -> Bus Creator/11  "states6"
  EventDetector/10 -> Bus Creator/10  "times5"
  EventDetector/9 -> Bus Creator/9  "states5"
  EventDetector/8 -> Bus Creator/8  "times4"
  EventDetector/7 -> Bus Creator/7  "states4"
  EventDetector/6 -> Bus Creator/6  "times3"
  EventDetector/5 -> Bus Creator/5  "states3"
  EventDetector/4 -> Bus Creator/4  "times2"
  EventDetector/3 -> Bus Creator/3  "states2"
  EventDetector/2 -> Bus Creator/2  "times1"
  EventDetector/1 -> Bus Creator/1  "states1"
  EventDetector/17 -> Terminator1/1
  EventGenerator1/1 -> Terminator2/1
  Bus Selector1/1 -> EventGenerator1/1  "<states 25>"
  Bus Selector1/2 -> EventGenerator1/2  "<times25>"
  Bus Selector1/3 -> EventGenerator1/3  "<states 26>"
  Bus Selector1/4 -> EventGenerator1/4  "<times26>"
  Bus Selector1/5 -> EventGenerator1/5  "<states 27>"
  Bus Selector1/6 -> EventGenerator1/6  "<times27>"
  Bus Selector1/7 -> EventGenerator1/7  "<states 28>"
  Bus Selector1/8 -> EventGenerator1/8  "<times28>"
  Bus Selector1/9 -> EventGenerator1/9  "<states 29>"
  Bus Selector1/10 -> EventGenerator1/10  "<times29>"
  Bus Selector1/11 -> EventGenerator1/11  "<states 30>"
  Bus Selector1/12 -> EventGenerator1/12  "<times30>"
  Bus Selector1/13 -> EventGenerator1/13  "<states 31>"
  Bus Selector1/14 -> EventGenerator1/14  "<times31>"
  Bus Selector1/15 -> EventGenerator1/15  "<states 32>"
  Bus Selector1/16 -> EventGenerator1/16  "<times32>"
  Bus Creator1/1 -> Bus Creator2/2  "CH24-31"
  EventDetector1/16 -> Bus Creator1/16  "times6"
  EventDetector1/15 -> Bus Creator1/15  "states6"
  EventDetector1/14 -> Bus Creator1/14  "times5"
  EventDetector1/13 -> Bus Creator1/13  "states5"
  EventDetector1/12 -> Bus Creator1/12  "times4"
  EventDetector1/11 -> Bus Creator1/11  "states4"
  EventDetector1/10 -> Bus Creator1/10  "times3"
  EventDetector1/9 -> Bus Creator1/9  "states3"
  EventDetector1/8 -> Bus Creator1/8  "times2"
  EventDetector1/7 -> Bus Creator1/7  "states2"
  EventDetector1/6 -> Bus Creator1/6  "times1"
  EventDetector1/5 -> Bus Creator1/5  "states1"
  EventDetector1/4 -> Bus Creator1/4  "times2"
  EventDetector1/3 -> Bus Creator1/3  "states2"
  EventDetector1/2 -> Bus Creator1/2  "times1"
  EventDetector1/1 -> Bus Creator1/1  "states1"
  EventDetector1/17 -> Terminator3/1  "states7"
  Bus Creator/1 -> Bus Creator2/1  "CH16-23"
  Bus Creator2/1 -> TSDin/1  "TSDIN"
